simulink model "project1_2021a"  (R2021a)
settings: Solver=ode2  StartTime=0.0  StopTime=7660  FixedStep=1  MaxStep=0.2  MinStep=1e-20  RelTol=1e-3
values from neighbouring files (symbols this model uses):
  A_F = 1.93    [init.m]
  C_0 = 0.015    [init.m]
  C_D = 0.35    [init.m]
  E_ess_max = E_batt_kW * 1000 * 3600    (= 7200000)    [init.m]
  eta_ess = 0.8    [init.m]
  g = 9.81    [init.m]
  G_diff = 0.268    [init.m]
  G_elec = 1    [init.m]
  grams_per_hr_to_gal_per_s = 9.778e-8    (= 9.778e-08)    [init.m]
  M_veh = M_glider + M_passengers + M_batt    (= 1976)    [init.m]
  meters_to_mi = 1/1609    (= 0.000621504039776)    [init.m]
  mi_per_hr_to_m_per_s = 0.44704    [init.m]
  r_wheel = 0.2794    [init.m]
  rho = 1.225    [init.m]
  SOC_init = 0.5    [init.m]
undefined symbols (not defined in the file or in its folder): eng_map, param, wltc
libraries: simulink x1
settings Model: Creator=wasynczu  LastModifiedBy=wasynczu
settings SolverCC: AlgebraicLoopSolver=TrustRegion
settings DebuggingCC: SFMachineParentedDataDiag=warning

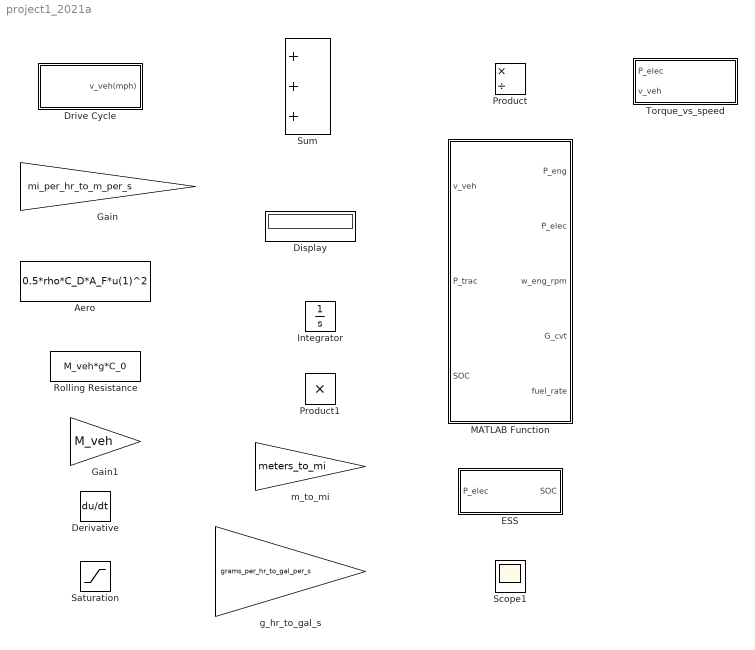
== system project1_2021a ==
  Aero : Fcn  Expr=0.5*rho*C_D*A_F*u(1)^2
  Derivative : Derivative
  Display : Display
  Drive Cycle : Subsystem  mask{schedule=wltc}
      mask prompts: schedule "drive schedule"
      mask init:
      | N=length(schedule(:,1));
  ESS : Subsystem  mask{E_max=E_ess_max, eta_ess=eta_ess}
      mask prompts: E_max "Maximum energy, J"; eta_ess "round-trip efficiency"
  Gain : Gain  Gain=mi_per_hr_to_m_per_s
  Gain1 : Gain  Gain=M_veh
  Integrator : Integrator
  MATLAB Function : MATLAB Function  TreatAsAtomicUnit=on
  Product : Product  Inputs=*/
  Product1 : Product
  Rolling Resistance : Constant  Value=M_veh*g*C_0
  Saturation : Saturate  UpperLimit=100  LowerLimit=0
  Scope1 : Scope
  Sum : Sum  Inputs=+++
  Torque_vs_speed : Subsystem
  g_hr_to_gal_s : Gain  Gain=grams_per_hr_to_gal_per_s
  m_to_mi : Gain  Gain=meters_to_mi

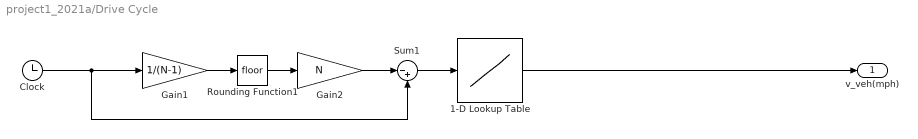
== system project1_2021a/Drive Cycle ==
  1-D Lookup Table : Lookup_n-D  NumberOfTableDimensions=1  BreakpointsForDimension1=schedule(:,1)  Table=schedule(:,2)  InterpMethod=Cubic spline  InternalRulePriority=Speed  RndMeth=Simplest  InputSameDT=on
  Clock : Clock
  Gain1 : Gain  Gain=1/(N-1)
  Gain2 : Gain  Gain=N
  Rounding Function1 : Rounding
  Sum1 : Sum  Inputs=|-+
  v_veh(mph) : Outport  VectorParamsAs1DForOutWhenUnconnected=off
  wires:
  Clock/1 -> Gain1/1, Sum1/2
  Sum1/1 -> 1-D Lookup Table/1
  Gain2/1 -> Sum1/1
  Rounding Function1/1 -> Gain2/1
  Gain1/1 -> Rounding Function1/1
  1-D Lookup Table/1 -> v_veh(mph)/1

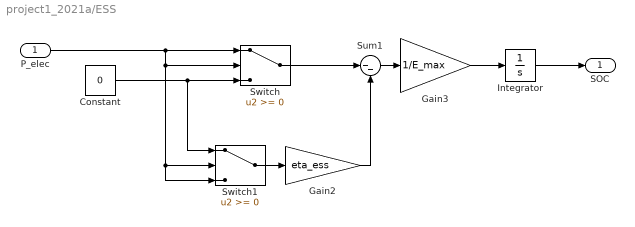
== system project1_2021a/ESS ==
  P_elec : Inport
  Constant : Constant  Value=0
  Gain2 : Gain  Gain=eta_ess
  Gain3 : Gain  Gain=1/E_max  OutDataTypeStr=fixdt('double', 'DataTypeOverride', 'Off')
  Integrator : Integrator  InitialCondition=SOC_init  LimitOutput=on  UpperSaturationLimit=1  LowerSaturationLimit=0
  Sum1 : Sum  Inputs=|--
  Switch : Switch  OutDataTypeStr=double
  Switch1 : Switch  OutDataTypeStr=double
  SOC : Outport  VectorParamsAs1DForOutWhenUnconnected=off
  wires:
  P_elec/1 -> Switch1/2, Switch1/3, Switch/2, Switch/1
  Gain3/1 -> Integrator/1
  Gain2/1 -> Sum1/2
  Switch1/1 -> Gain2/1
  Sum1/1 -> Gain3/1
  Switch/1 -> Sum1/1
  Constant/1 -> Switch1/1, Switch/3
  Integrator/1 -> SOC/1

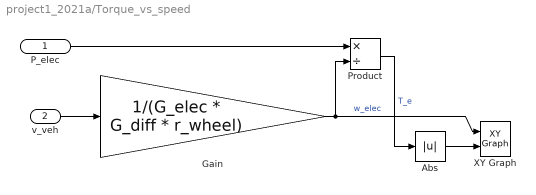
== system project1_2021a/Torque_vs_speed ==
  P_elec : Inport
  v_veh : Inport  Port=2
  Abs : Abs
  Gain : Gain  Gain=1/(G_elec * G_diff * r_wheel)
  Product : Product  Inputs=*/
  XY Graph : simulink/Sinks/XY Graph  xmin=0  xmax=500  ymin=0  ymax=700  st=-1
  wires:
  P_elec/1 -> Product/1
  Product/1 -> Abs/1  "T_e"
  v_veh/1 -> Gain/1
  Gain/1 -> XY Graph/1, Product/2  "w_elec"
  Abs/1 -> XY Graph/2

== matlab function project1_2021a/MATLAB Function ==
  data: v_veh input; P_eng output; P_trac input; SOC input; P_elec output; w_eng_rpm output; G_cvt output; fuel_rate output; param parameter; eng_map parameter
function [P_eng, P_elec, w_eng_rpm, G_cvt, fuel_rate] = fcn(v_veh, P_trac, SOC, param, eng_map)
%#codegen
%inputs:
    % v_veh, m/s
    % P_trac, W
    % SOC
    % param, structure of parameters
    % eng_map

% outputs:
    %   P_gen, P_elec in W
    %   w_eng_rpm, rpm
    %   G_cvt (cvt ratio)
    %   Fuel rate, grams/hr

v_veh_min = param.v_veh_min;    % minimum vehicle speed for engine to stay engaged, in m/s
P_eng_min = param.P_eng_min;    % minimum engine power in W
P_eng_max = param.P_eng_max ;   % maximum engine power
G_cvt_min = param.G_cvt_min;    % minimum cvt  ratio
G_diff = param.G_diff;          % differential gear ratio
r_wheel = param.r_wheel;        % wheel radius in m

if (v_veh < v_veh_min)  % disengage clutch, idle engine, electric propulsion
   P_elec = P_trac;
   P_eng = 0;
   fuel_rate = 0; % g/hr;
   w_eng_rpm = 1000; % rpm
   G_cvt = G_cvt_min;
   return  
end

% if here, v_veh > v_veh_min
if(P_trac < P_eng_min)   % clutch engaged but engine idling
   P_elec = P_trac;
   fuel_rate = 0;
   P_eng = 0;
   w_eng_rpm =  1000; % rpm
   w_eng = w_eng_rpm * pi / 30; % rad/s
   % set G_cvt so engine speed is 1000 rpm
   G_cvt = v_veh/G_diff/w_eng/r_wheel;
   return     
end

if(P_trac > P_eng_max) % high-speed boost
   P_elec = P_trac - P_eng_max;
   P_eng = P_eng_max;
   bsfc = interp1(eng_map(:,2), eng_map(:,3), P_eng/1000, 'pchip', 'extrap');
   fuel_rate = bsfc*P_eng/1000; % grams/hr
   w_eng_rpm = interp1(eng_map(:,2), eng_map(:,1), P_eng/1000, 'pchip', 'extrap');
   w_eng = w_eng_rpm * pi / 30; % convert to rad/s
   G_cvt =  v_veh/r_wheel/G_diff/w_eng; % required CVT ratio
   return   
end

% if here, v_veh > v_veh_min and P_eng_min < P_trac < P_eng_max
% try to get SOC back to 0.5

P_elec = 4000*sign(SOC - 0.5); 
P_eng = P_trac - P_elec;


if(P_eng < P_eng_min) 
   % clutch engaged, but no fuel
   P_eng = 0;
   P_elec = P_trac;
   fuel_rate = 0;
   w_eng_rpm = 1000;
   w_eng = w_eng_rpm * 2 * pi / 60; % in rad/s
   % set G_cvt so engine speed is 1000 rpm
   G_cvt = v_veh/G_diff/w_eng/r_wheel;
   return
end

if(P_eng > P_eng_max)
    P_eng = P_eng_max;
    P_elec = P_trac - P_eng_max;
end

bsfc = interp1(eng_map(:,2), eng_map(:,3), P_eng/1000, 'pchip', 'extrap');
fuel_rate = bsfc*P_eng/1000; % grams/hr

w_eng_rpm = interp1(eng_map(:,2), eng_map(:,1), P_eng/1000, 'pchip', 'extrap');
if(w_eng_rpm < 1000)
    w_eng_rpm = 1000;
end
w_eng = w_eng_rpm * pi / 30;  % convert to rad/s
G_cvt =  v_veh/r_wheel/G_diff/w_eng;

if (G_cvt < G_cvt_min) % set G_cvt = G_cvt_min, recalculate w_eng, P_eng, and P_elec
   G_cvt = G_cvt_min;
   w_eng = v_veh/G_diff/r_wheel/G_cvt;
   w_eng_rpm = w_eng*30/pi;  % in rpm
   P_eng = 1000*interp1(eng_map(:,1), eng_map(:,2), w_eng, 'pchip', 'extrap'); % in W
   if(P_eng < 0)
       P_eng = 0;
   end
   P_elec = P_trac - P_eng;
   bsfc = interp1(eng_map(:,1), eng_map(:,3), w_eng, 'pchip', 'extrap');
   fuel_rate = bsfc*P_eng/1000; % grams/hr
 end
